simulink model "aie_hls"  (R2021a)
settings: Solver=VariableStepAuto  StartTime=0.0  StopTime=4000  RelTol=1e-3
InitFcn:
  | %xmcCheckSlxPath(bdroot);
  | input = readcomplexdata('./sw/input.h');
undefined symbols (not defined in the file): xc7vx485tffg1157
libraries: aieBasic x2, aieUtilities x2, simulink x1, vmcUtilities x1, dspsrcs4 x1, hlsBasic x1
settings Model: Creator=abehbood  LastModifiedBy=abehbood
settings SolverCC: AlgebraicLoopSolver=TrustRegion
settings DebuggingCC: SFMachineParentedDataDiag=warning
settings SFSimCC: CustomCodeUndefinedFunction=UseInterfaceOnly

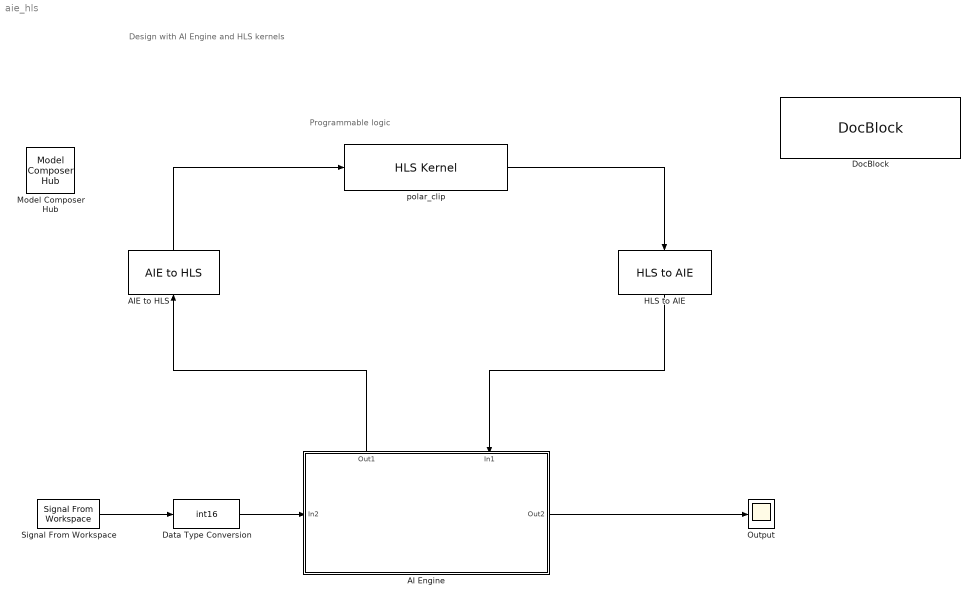
== system aie_hls ==
  note: Programmable logic
  note: Design with AI Engine and HLS kernels
  AI Engine : Subsystem
      settings: PortSchema="{\"entries\":[{\"content\":{\"sides\":[{\"content\":{\"connectorIds\":[\"In1\"]},\"type\":\"ConnectorPlacement.EquallySpacedRectSide\",\"uuid\":\"4c582470-6e07-4cf2-89ba-1d9148c6c342\"},{\"content\":{\"connectorIds\":[\"Out1\"],\"side\":\"RIGHT\"},\"type\":\"ConnectorPlacement.EquallySpacedRectSide\",\"uuid\":\"202127b6-913d-45d6-97d3-63d531af815e\"},{\"content\":{\"connectorIds\":[\"Out2\",\"In2\"],\"side\":\"TOP\"},\"type\":\"ConnectorPlacement.EquallySpacedRectSide\",\"uuid\":\"5b5cfc98-70f5-4b9e-bee7-2ee5eb3017f9\"}]},\"type\":\"ConnectorPlacement.EquallySpacedConnector\",\"uuid\":\"3aebc8b4-6a22-4c89-86c8-92d2be0437af\"}],\"packageUris\":[\"http://schema.mathworks.com/mf0/Connector/R2020b\"],\"version\":\"1.0\"}"
  AIE to HLS : aieUtilities/AIE to HLS  OutputType=ap_axis<32,0,0,0>  OutputSize=256
  Data Type Conversion : DataTypeConversion  OutDataTypeStr=int16
  DocBlock : simulink/Model-Wide Utilities/DocBlock  DocumentType=Text  mask(DocBlock){}
      content=|
      | ///////////////////////////////////////////////////////////////////////////
      | // Copyright 2021 Xilinx
      | //
      | // Licensed under the Apache License, Version 2.0 (the "License");
      | // you may not use this file except in compliance with the License.
      | // You may obtain a copy of the License at
      | //
      | // http://www.apache.org/licenses/LICENSE-2.0
      | //
      | // Unless required by applicable law or agreed to in writing, software
      | // distributed under the License is distributed on an "AS IS" BASIS,
      | // WITHOUT WARRANTIES OR CONDITIONS OF ANY KIND, either express or implied.
      | // See the License for the specific language governing permissions and
      | // limitations under the License.
      | ///////////////////////////////////////////////////////////////////////////
      mask Display:
      | xmcDrawBlockIcon();
      | disp(['{\fontsize{10pt}(c) Copyright 2021' ' Xilinx, Inc.}\newline \newline '],'texmode','on');
      | disp('{\fontsize{10pt}Licensed under the Apache License 2.0}','texmode','on');
      | disp('\newline \newline \newline{\fontsize{10pt}Double Click for Copyright Notice}','texmode','on');
  HLS to AIE : aieUtilities/HLS to AIE  OutputType=cint16  OutputSize=256
  Model Composer Hub : vmcUtilities/Model Composer Hub  CodeGeneration=off  SubsystemName=AI Engine  TargetDirectory=./code_xrt  ExportType=AI Engines  IpVendor=xilinx.com  IpLibrary=hls  IpVersion=1.0  IpHWLanguage=Verilog  AieCompilerOptions={}  CreateTestbench=on  TestbenchStackSize=10  RunAieSim=on  AieSimTimeout=50000  RunAieSimProfiling=off  LaunchVitisAnalyzer=off  PlotOutput=off  RunX86Sim=off  X86SimTimeout=10  GenHwImage=off  PlatformType=Not Specified  HwValidationTarget=hw  ProjDevice=xc7vx485tffg1157-1  ProjDevicePart=xc7vx485tffg1157-1  SamplePeriod=-1  ClockFrequency=200  DataPathParallelism=1
  Output : Scope
  Signal From Workspace : dspsrcs4/Signal From Workspace  X=input  Ts=1  nsamps=128  OutputAfterFinalValue=Setting to zero  ignoreOrWarnInputAndFrameLengths=off  OutputFrames=off
  polar_clip : hlsBasic/HLS Kernel  PortNames={}  PortSerializedTypes={}  FunctionTemplateParamNames={}  FunctionTemplateParamKinds={}  FunctionTemplateParamTypes={}  FunctionTemplateParamValues={}  PortSynchronicities={'auto'; 'auto'}  PortSignalSizes={0.000000000000000000e+00; 2.560000000000000000e+02}  FunctionTemplateParams={}  FunctionTemplateParamsEnables={}  FunctionTemplateParamsVisible=off  FunctionDeclTypeOptions=C[1 1]@t7@<empty>  PortAttributesTable={ 'Input', 'in_sample', 'hls::stream< hls::axis< ap_int< 32 >, 0, 0, 0 >, 0 > &', '', ''; 'Output', 'out_sample', 'hls::stream< hls::axis< ap_int< 32 >, 0, 0, 0 >, 0 > &', '', '256' }  PortAttributesEnablement={'off', 'off', 'off', 'off', 'off';'off', 'off', 'off', 'off', 'on'}  SampleTime=-1  PortDirectionTable={ 'in_sample', 'hls::stream< hls::axis< ap_int< 32 >, 0, 0, 0 >, 0 > &', 'Input'; 'out_sample', 'hls::stream< hls::axis< ap_int< 32 >, 0, 0, 0 >, 0 > &', 'Output' }  PortDirectionTabVisible=on  ArgDirections={1.000000000000000000e+00; 2.000000000000000000e+00}  FunctionIndex=1  FormalArgDecls={'hls::stream< hls::axis< ap_int< 32 >, 0, 0, 0 >, 0 > & in_sample', 'hls::stream< hls::axis< ap_int< 32 >, 0, 0, 0 >, 0 > & out_sample'}  SimLibPath=''  FunctionTabVisible=on  FunctionDescription=void polar_clip(hls::stream< hls::axis< ap_int< 32 >, 0, 0, 0 >, 0 > & in_sample, hls::stream< hls::axis< ap_int< 32 >, 0, 0, 0 >, 0 > & out_sample)  KernelHeaderFile=src/hls_kernels.h  KernelFunction=polar_clip  KernelFunctionSelect=<empty>  KernelSourceFile=src/polar_clip.cpp  KernelSearchPaths={}  PreProcOptions={}  blockJsonConstraints=[]  deprecateConstraints=0
  wires:
  polar_clip/1 -> HLS to AIE/1
  Signal From Workspace/1 -> Data Type Conversion/1
  AIE to HLS/1 -> polar_clip/1
  HLS to AIE/1 -> AI Engine/2(In1)
  Data Type Conversion/1 -> AI Engine/1(In2)
  AI Engine/2(Out1) -> AIE to HLS/1
  AI Engine/1(Out2) -> Output/1

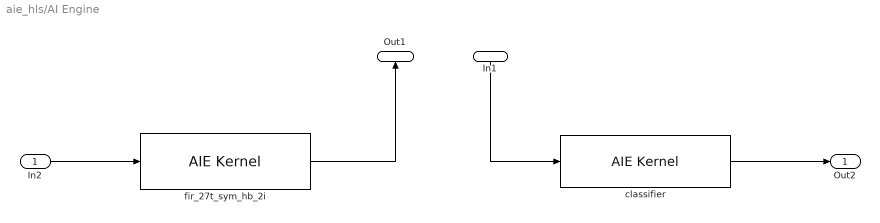
== system aie_hls/AI Engine ==
  In2 : Inport
  In1 : Inport  Port=2
  classifier : aieBasic/AIE Kernel  KernelAllAttrs=s[12;12;9;9;19;14;21;23;24;21;12;24;26;26;26;27;28;9;21;23;23;23;24;25;14;19;19;29]@FunctionNameDeclFileNamePortNamesPortTypesPortSerializedTypesPortDirectionsPortWindowSizeEnablesPortWindowMarginEnablesPortSynchronicityEnablesPortSignalSizeEnablesFunctionDeclFunctionTemplateSpecKindFunctionTemplateParamNamesFunctionTemplateParamKindsFunctionTemplateParamTypesFunctionTemplateParamValuesFunctionTemplateParamEnablesClassDeclClassTemplateSpecKindClassTemplateParamNamesClassTemplateParamKindsClassTemplateParamTypesClassTemplateParamValuesClassTemplateParamEnablesClassCtorDeclsClassCtorParamNamesClassCtorParamTypesClassCtorParamSerializedTypes[1 1]@C[28 1]@t10@classifiert19@../../src/kernels.hC[2 1]@t5@inputt6@outputC[2 1]@t21@input_stream_cint16 *t21@output_window_int32 *C[2 1]@t33@{P{Tinput_stream{1{t{Scint16}}}}}t31@{P{Toutput_window{1{t{Bi32}}}}}C[2 1]@t5@inputt6@outputC[2 1]@l0@l1@C[2 1]@l0@l0@C[2 1]@l0@l1@C[2 1]@l0@l0@t74@void classifier(input_stream_cint16 * input, output_window_int32 * output)t4@nonee[0 1]@e[0 1]@e[0 1]@e[0 1]@e[0 1]@nne[0 1]@e[0 1]@e[0 1]@e[0 1]@e[0 1]@e[0 1]@e[0 1]@e[0 1]@e[0 1]@  PortNames={'input'; 'output'}  PortSerializedTypes={'{P{Tinput_stream{1{t{Scint16}}}}}'; '{P{Toutput_window{1{t{Bi32}}}}}'}  PortWindowSizes={0.000000000000000000e+00; 2.560000000000000000e+02}  PortWindowMargins={0.000000000000000000e+00; 0.000000000000000000e+00}  PortSynchronicities={'auto'; 'sync'}  PortSignalSizes={0.000000000000000000e+00; 0.000000000000000000e+00}  FunctionTemplateSpecKind=none  FunctionTemplateParamNames={}  FunctionTemplateParamKinds={}  FunctionTemplateParamTypes={}  FunctionTemplateParamValues={}  FunctionIndex=1  FunctionTabVisible=on  FunctionTemplateParamsVisible=off  FunctionDeclTypeOptions=C[1 1]@t74@void classifier(input_stream_cint16 * input, output_window_int32 * output)  FunctionDecl=void classifier(input_stream_cint16 * input, output_window_int32 * output)  FunctionTemplateParams={}  FunctionTemplateParamsEnables={}  PortAttrs={ 'Input', 'input', 'input_stream_cint16 *', '', '', '', ''; 'Output', 'output', 'output_window_int32 *', '256', '', 'sync', '' }  PortAttrsEnables={'off', 'off', 'off', 'off', 'off', 'off', 'off';'off', 'off', 'off', 'on', 'off', 'on', 'off'}  SampleTime=-1  KernelHeaderFile=src/kernels.h  KernelFunction=classifier  KernelSourceFile=src/kernels/classifiers/classify.cc  KernelSearchPaths={}  PreProcOptions={}  CoreRuntimeRatio=0.9  KernelLocSpec=off  ColRowLocation=[0 0]  blockJsonConstraints="{\"type\":\"constraint\",\"constraintType\":\"coreUtilization\",\"sid\":\"3\",\"lhs\":{\"type\":\"runtimeRatio\",\"args\":{\"type\":\"kernel\",\"name\":\"aie_hls/AI Engine/classifier\",\"sid\":\"3\"}},\"rhs\":{\"type\":\"evaluable\",\"expr\":\"0.9\",\"value\":0.9},\"equality\":true}"  deprecateConstraints=1
  fir_27t_sym_hb_2i : aieBasic/AIE Kernel  KernelAllAttrs=s[12;12;9;9;19;14;21;23;24;21;12;24;26;26;26;27;28;9;21;23;23;23;24;25;14;19;19;29]@FunctionNameDeclFileNamePortNamesPortTypesPortSerializedTypesPortDirectionsPortWindowSizeEnablesPortWindowMarginEnablesPortSynchronicityEnablesPortSignalSizeEnablesFunctionDeclFunctionTemplateSpecKindFunctionTemplateParamNamesFunctionTemplateParamKindsFunctionTemplateParamTypesFunctionTemplateParamValuesFunctionTemplateParamEnablesClassDeclClassTemplateSpecKindClassTemplateParamNamesClassTemplateParamKindsClassTemplateParamTypesClassTemplateParamValuesClassTemplateParamEnablesClassCtorDeclsClassCtorParamNamesClassCtorParamTypesClassCtorParamSerializedTypes[1 1]@C[28 1]@t17@fir_27t_sym_hb_2it19@../../src/kernels.hC[2 1]@t7@inputcbt8@outputcbC[2 1]@t21@input_window_cint16 *t22@output_window_cint16 *C[2 1]@t33@{P{Tinput_window{1{t{Scint16}}}}}t34@{P{Toutput_window{1{t{Scint16}}}}}C[2 1]@t5@inputt6@outputC[2 1]@l1@l1@C[2 1]@l1@l0@C[2 1]@l1@l1@C[2 1]@l0@l0@t86@void fir_27t_sym_hb_2i(input_window_cint16 * inputcb, output_window_cint16 * outputcb)t4@nonee[0 1]@e[0 1]@e[0 1]@e[0 1]@e[0 1]@nne[0 1]@e[0 1]@e[0 1]@e[0 1]@e[0 1]@e[0 1]@e[0 1]@e[0 1]@e[0 1]@  PortNames={'inputcb'; 'outputcb'}  PortSerializedTypes={'{P{Tinput_window{1{t{Scint16}}}}}'; '{P{Toutput_window{1{t{Scint16}}}}}'}  PortWindowSizes={1.280000000000000000e+02; 2.560000000000000000e+02}  PortWindowMargins={1.600000000000000000e+01; 0.000000000000000000e+00}  PortSynchronicities={'sync'; 'sync'}  PortSignalSizes={0.000000000000000000e+00; 0.000000000000000000e+00}  FunctionTemplateSpecKind=none  FunctionTemplateParamNames={}  FunctionTemplateParamKinds={}  FunctionTemplateParamTypes={}  FunctionTemplateParamValues={}  FunctionIndex=1  FunctionTabVisible=on  FunctionTemplateParamsVisible=off  FunctionDeclTypeOptions=C[1 1]@t86@void fir_27t_sym_hb_2i(input_window_cint16 * inputcb, output_window_cint16 * outputcb)  FunctionDecl=void fir_27t_sym_hb_2i(input_window_cint16 * inputcb, output_window_cint16 * outputcb)  FunctionTemplateParams={}  FunctionTemplateParamsEnables={}  PortAttrs={ 'Input', 'inputcb', 'input_window_cint16 *', '128', '16', 'sync', ''; 'Output', 'outputcb', 'output_window_cint16 *', '256', '', 'sync', '' }  PortAttrsEnables={'off', 'off', 'off', 'on', 'on', 'on', 'off';'off', 'off', 'off', 'on', 'off', 'on', 'off'}  SampleTime=-1  KernelHeaderFile=src/kernels.h  KernelFunction=fir_27t_sym_hb_2i  KernelSourceFile=src/kernels/interpolators/hb27_2i.cc  KernelSearchPaths={}  PreProcOptions={}  CoreRuntimeRatio=0.9  KernelLocSpec=off  ColRowLocation=[0 0]  blockJsonConstraints="{\"type\":\"constraint\",\"constraintType\":\"coreUtilization\",\"sid\":\"1\",\"lhs\":{\"type\":\"runtimeRatio\",\"args\":{\"type\":\"kernel\",\"name\":\"aie_hls/AI Engine/fir_27t_sym_hb_2i\",\"sid\":\"1\"}},\"rhs\":{\"type\":\"evaluable\",\"expr\":\"0.9\",\"value\":0.9},\"equality\":true}"  deprecateConstraints=1
  Out2 : Outport  VectorParamsAs1DForOutWhenUnconnected=off
  Out1 : Outport  Port=2  VectorParamsAs1DForOutWhenUnconnected=off
  wires:
  fir_27t_sym_hb_2i/1 -> Out1/1
  In2/1 -> fir_27t_sym_hb_2i/1
  In1/1 -> classifier/1
  classifier/1 -> Out2/1
